simulink model "chap9_2sim"  (Simulink 3.00)
settings: Solver=ode4  SolverMode=SingleTasking  StartTime=0.0  StopTime=6  FixedStep=0.001  RelTol=1e-3
settings Model: LastModifiedBy=liu

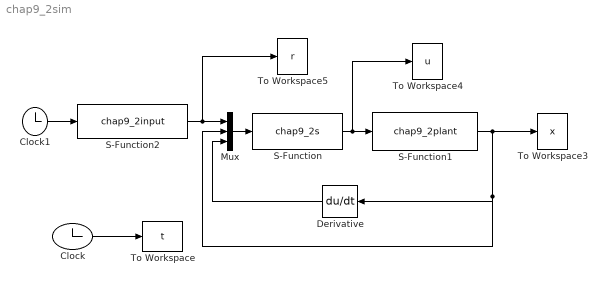
== system chap9_2sim ==
  Clock : Clock
  Clock1 : Clock
      settings: DisplayTime=off  Decimation=10
  Derivative : Derivative  Orientation=left
  Mux : Mux  Inputs=3
  S-Function : S-Function  FunctionName=chap9_2s  PortCounts=[]  SFunctionModules=''
  S-Function1 : S-Function  FunctionName=chap9_2plant  PortCounts=[]  SFunctionModules=''
  S-Function2 : S-Function  FunctionName=chap9_2input  PortCounts=[]  SFunctionModules=''
  To Workspace : ToWorkspace  VariableName=t  SampleTime=-1  SaveFormat=Matrix
  To Workspace3 : ToWorkspace  VariableName=x  SampleTime=-1  SaveFormat=Matrix
  To Workspace4 : ToWorkspace  VariableName=u  SampleTime=-1  SaveFormat=Matrix
  To Workspace5 : ToWorkspace  VariableName=r  SampleTime=-1  SaveFormat=Matrix
  wires:
  Clock1/1 -> S-Function2/1
  Mux/1 -> S-Function/1
  S-Function1/1 -> To Workspace3/1, Mux/2, Derivative/1
  Clock/1 -> To Workspace/1
  S-Function/1 -> S-Function1/1, To Workspace4/1
  S-Function2/1 -> Mux/1, To Workspace5/1
  Derivative/1 -> Mux/3
